simulink model "quadrotorv3"  (R2019a)
settings: Solver=ode4  StartTime=0.0  StopTime=10  FixedStep=0.01  RelTol=1e-3  EnableMultiTasking=on
model workspace: external: MATLAB File C:\Users\zxz\Desktop\matlab\msimscape\quadrotorv3\quadrotorv3_DataFile.m (data not in the file)
undefined symbols (not defined in the file or in its folder): magnitude, smiData, X, Y, Z
libraries: sm_lib x84, nesl_utility x35, sharedtransform x1
(part 3 of 3)

== matlab function quadrotorv3/control/eang  ==
  data: eang output size=3; deang output size=3; angd input size=3; dangd input size=3; ang input size=3; dang input size=3
function [eang,deang] = fcn(angd,dangd,ang,dang)

eang  = angd  - ang;
deang = dangd - dang;

== matlab function quadrotorv3/control/ep ==
  data: ep output; dep output; pd input; dpd input; p input; dp input
function [ep,dep] = fcn(pd,dpd,p,dp)

ep  = pd-p;
dep = dpd-dp;
